simulink model "Model_ar42"  (R2020b)
settings: Solver=VariableStepAuto  StartTime=0.0  StopTime=120  RelTol=1e-3
libraries: SignalEditorBlockLib x1, simulink x1
settings Model: Creator=Stend  LastModifiedBy=Stend

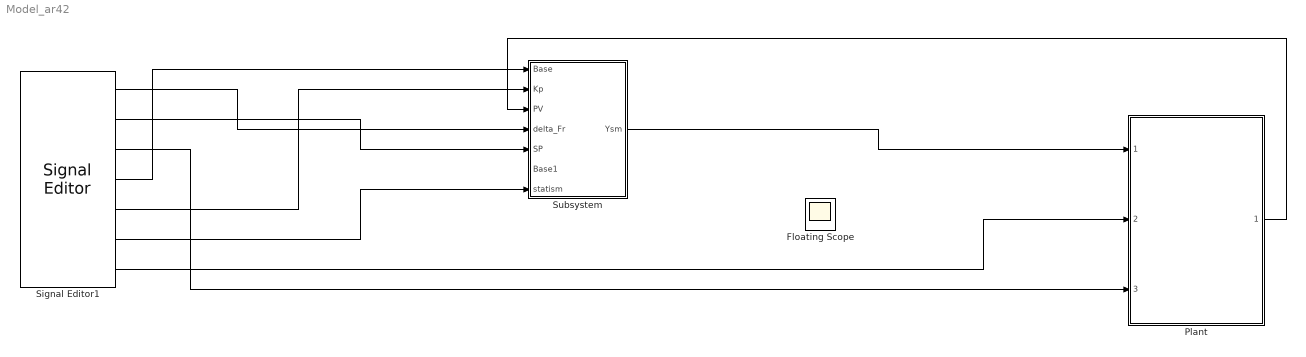
== system Model_ar42 ==
  Floating Scope : Scope
      settings: Floating=on
  Plant : Subsystem  ReferencedSubsystem=PlantPModel
  Signal Editor1 : SignalEditorBlockLib/Signal Editor  FileName=Psp_deltaFr.mat  ActiveScenario=Scenario1  ActiveSignal=delta_Fr  IsBus=off  OutputBusObjectStr=Bus: BusObject  SampleTime=0  Interpolate=off  ZeroCross=off  OutputAfterFinalValue=Setting to zero  Unit=inherit  PreserveSignalName=on
  Subsystem : Subsystem
  wires:
  Plant/1 -> Subsystem/3(PV)
  Signal Editor1/3 -> Plant/3
  Signal Editor1/7 -> Plant/2
  Subsystem/1(Ysm) -> Plant/1
  Signal Editor1/4 -> Subsystem/1(Base)
  Signal Editor1/5 -> Subsystem/2(Kp)
  Signal Editor1/1 -> Subsystem/4(delta_Fr)
  Signal Editor1/2 -> Subsystem/5(SP)
  Signal Editor1/6 -> Subsystem/7(statism)

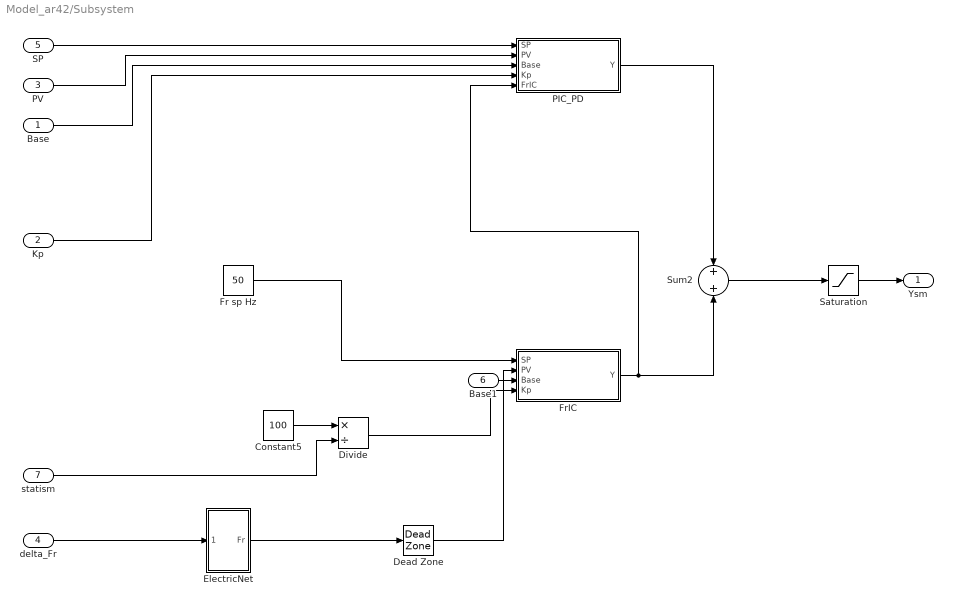
== system Model_ar42/Subsystem ==
  Base : Inport
  Kp : Inport  Port=2
  PV : Inport  Port=3
  delta_Fr : Inport  Port=4
  SP : Inport  Port=5
  Base1 : Inport  Port=6
  statism : Inport  Port=7
  Constant5 : Constant  Value=100
  Dead Zone : DeadZone  LowerValue=-0.02  UpperValue=0.02  SaturateOnIntegerOverflow=on
  Divide : Product  Inputs=*/
  ElectricNet : Subsystem
  Fr sp Hz : Constant  Value=50
  FrIC : Subsystem  TreatAsAtomicUnit=on
  PIC_PD : Subsystem  TreatAsAtomicUnit=on
  Saturation : Saturate  UpperLimit=100  LowerLimit=0
  Sum2 : Sum  Inputs=+|+  InputSameDT=on  SaturateOnIntegerOverflow=on  OutDataTypeStr=Inherit: Same as first input
  Ysm : Outport
  wires:
  Dead Zone/1 -> FrIC/2(PV)
  PIC_PD/1(Y) -> Sum2/1
  FrIC/1(Y) -> Sum2/2, PIC_PD/5(FrIC)
  SP/1 -> PIC_PD/1(SP)
  Constant5/1 -> Divide/1
  Divide/1 -> FrIC/4(Kp)
  Sum2/1 -> Saturation/1
  ElectricNet/1(Fr) -> Dead Zone/1
  Fr sp Hz/1 -> FrIC/1(SP)
  PV/1 -> PIC_PD/2(PV)
  Kp/1 -> PIC_PD/4(Kp)
  delta_Fr/1 -> ElectricNet/1(delta_Fr)
  Base/1 -> PIC_PD/3(Base)
  statism/1 -> Divide/2
  Saturation/1 -> Ysm/1
  Base1/1 -> FrIC/3(Base)

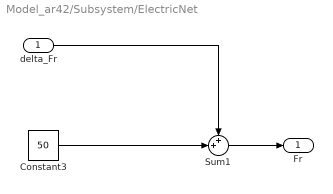
== system Model_ar42/Subsystem/ElectricNet ==
  delta_Fr : Inport
  Constant3 : Constant  Value=50
  Sum1 : Sum  Inputs=++|  InputSameDT=on  SaturateOnIntegerOverflow=on  OutDataTypeStr=Inherit: Same as first input
  Fr : Outport
  wires:
  Sum1/1 -> Fr/1
  Constant3/1 -> Sum1/2
  delta_Fr/1 -> Sum1/1

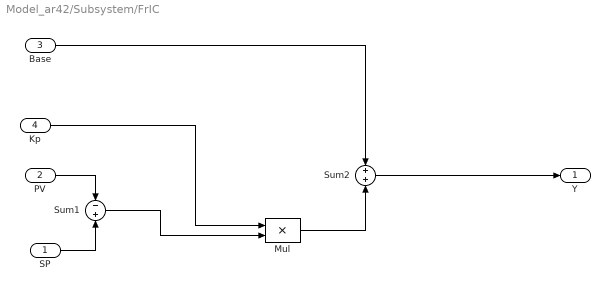
== system Model_ar42/Subsystem/FrIC ==
  SP : Inport
  PV : Inport  Port=2
  Base : Inport  Port=3
  Kp : Inport  Port=4
  Mul : Product  InputSameDT=on  SaturateOnIntegerOverflow=on  OutDataTypeStr=Inherit: Same as first input
  Sum1 : Sum  Inputs=-+  InputSameDT=on  SaturateOnIntegerOverflow=on  OutDataTypeStr=Inherit: Same as first input
  Sum2 : Sum  InputSameDT=on  SaturateOnIntegerOverflow=on  OutDataTypeStr=Inherit: Same as first input
  Y : Outport  OutputWhenDisabled=reset  InitialOutput=0  VectorParamsAs1DForOutWhenUnconnected=off
  wires:
  Kp/1 -> Mul/1
  Base/1 -> Sum2/1
  Sum2/1 -> Y/1
  PV/1 -> Sum1/1
  SP/1 -> Sum1/2
  Sum1/1 -> Mul/2
  Mul/1 -> Sum2/2

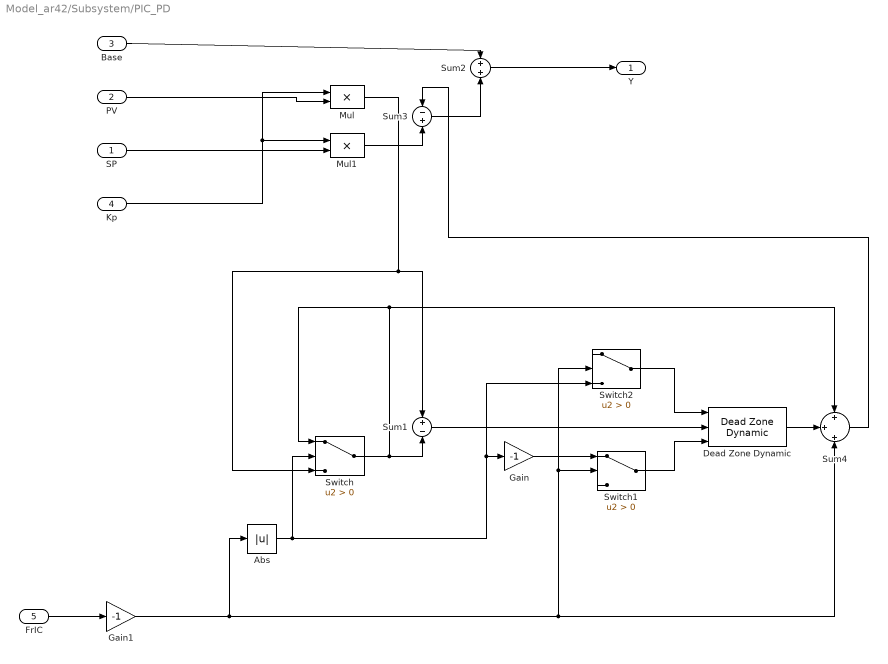
== system Model_ar42/Subsystem/PIC_PD ==
  SP : Inport
  PV : Inport  Port=2
  Base : Inport  Port=3
  Kp : Inport  Port=4
  FrIC : Inport  Port=5
  Abs : Abs
  Dead Zone Dynamic : simulink/Discontinuities/Dead Zone Dynamic
      settings: SourceProductBaseCode=SL
  Gain : Gain  Gain=-1
  Gain1 : Gain  Gain=-1
  Mul : Product  InputSameDT=on  SaturateOnIntegerOverflow=on  OutDataTypeStr=Inherit: Same as first input
  Mul1 : Product  InputSameDT=on  SaturateOnIntegerOverflow=on  OutDataTypeStr=Inherit: Same as first input
  Sum1 : Sum  Inputs=+-  InputSameDT=on  SaturateOnIntegerOverflow=on  OutDataTypeStr=Inherit: Same as first input
  Sum2 : Sum  InputSameDT=on  SaturateOnIntegerOverflow=on  OutDataTypeStr=Inherit: Same as first input
  Sum3 : Sum  Inputs=-+  InputSameDT=on  SaturateOnIntegerOverflow=on  OutDataTypeStr=Inherit: Same as first input
  Sum4 : Sum  Inputs=+|+|+  InputSameDT=on  SaturateOnIntegerOverflow=on  OutDataTypeStr=Inherit: Same as first input
  Switch : Switch  Criteria=u2 > Threshold
  Switch1 : Switch  Criteria=u2 > Threshold
  Switch2 : Switch  Criteria=u2 > Threshold
  Y : Outport  OutputWhenDisabled=reset  InitialOutput=0  VectorParamsAs1DForOutWhenUnconnected=off
  wires:
  Kp/1 -> Mul/1, Mul1/1
  Base/1 -> Sum2/1
  Sum2/1 -> Y/1
  SP/1 -> Mul1/2
  PV/1 -> Mul/2
  Mul1/1 -> Sum3/2
  Sum3/1 -> Sum2/2
  Dead Zone Dynamic/1 -> Sum4/2
  Switch2/1 -> Dead Zone Dynamic/1
  Mul/1 -> Switch/3, Sum1/1
  Sum4/1 -> Sum3/1
  Gain/1 -> Switch1/1
  Sum1/1 -> Dead Zone Dynamic/2
  Gain1/1 -> Abs/1, Switch1/2, Switch2/2, Sum4/3
  Abs/1 -> Switch/2, Switch2/3, Gain/1
  Switch1/1 -> Dead Zone Dynamic/3
  Switch/1 -> Sum1/2, Sum4/1, Switch/1
  FrIC/1 -> Gain1/1
